simulink model "MatrixModel"  (R2018b)
settings: Solver=ode45  StartTime=0.0  StopTime=10.0  RelTol=1e-3  EnableMultiTasking=on
settings Model: Creator=sz609516  LastModifiedBy=fhu-eba
settings DataIOCC: LimitDataPoints=on  SaveFormat=Array
settings OptimizationCC: LifeSpan=inf
settings DebuggingCC: UnderspecifiedInitializationDetection=Classic  MergeDetectMultiDrivingBlocksExec=none  SolverPrmCheckMsg=warning  StateNameClashWarn=warning  SFUnexpectedBacktrackingDiag=warning  SFNoUnconditionalDefaultTransitionDiag=warning
settings HardwareCC: ProdBitPerPointer=32  ProdBitPerSizeT=32  ProdBitPerPtrDiffT=32  ProdLargestAtomicFloat=None  ProdIntDivRoundTo=Undefined  ProdEndianess=Unspecified  ProdWordSize=32  ProdHWDeviceType=32-bit Generic
settings ModelReferenceCC: PropagateSignalLabelsOutOfModel=off
settings SFSimCC: SimUseLocalCustomCode=off
settings RTWCC: RTWUseLocalCustomCode=off
settings CodeAppCC: StateflowObjectComments=on
settings GRTTargetCC: TargetLangStandard=C89/C90 (ANSI)  GeneratePreprocessorConditionals=Disable all
settings ConfigComp: CovMetricSettings=dw  CovHtmlReporting=on  CovSaveCumulativeToWorkspaceVar=on  CovSaveSingleToWorkspaceVar=on  CovExternalEMLEnable=off

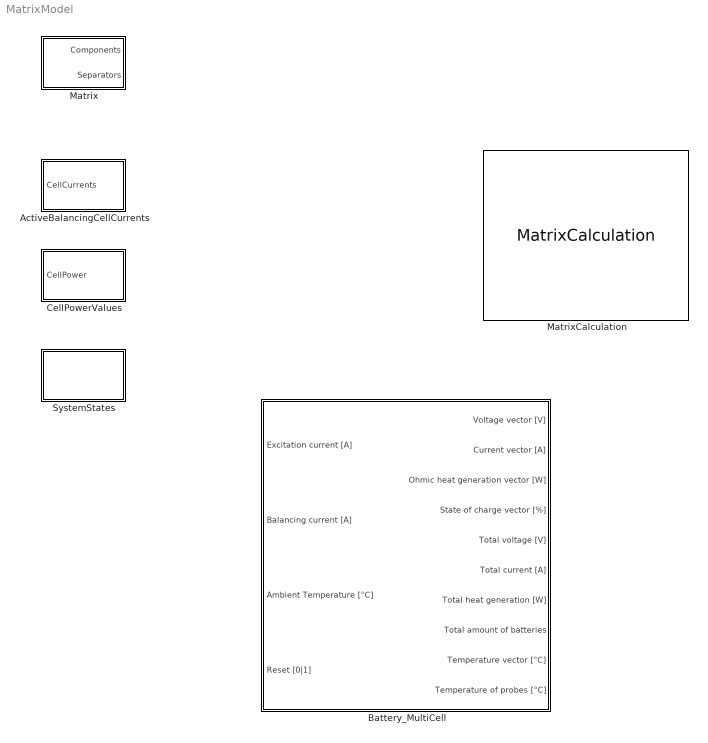
== system MatrixModel ==
  ActiveBalancingCellCurrents : Subsystem
  Battery_MultiCell : Subsystem
  CellPowerValues : Subsystem
  Matrix : Subsystem
  MatrixCalculation : S-Function  FunctionName=MatrixCalculation  SFunctionDeploymentMode=off  EnableBusSupport=off
  SystemStates : Subsystem

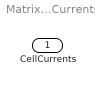
== system MatrixModel/ActiveBalancingCellCurrents ==
  CellCurrents : Inport

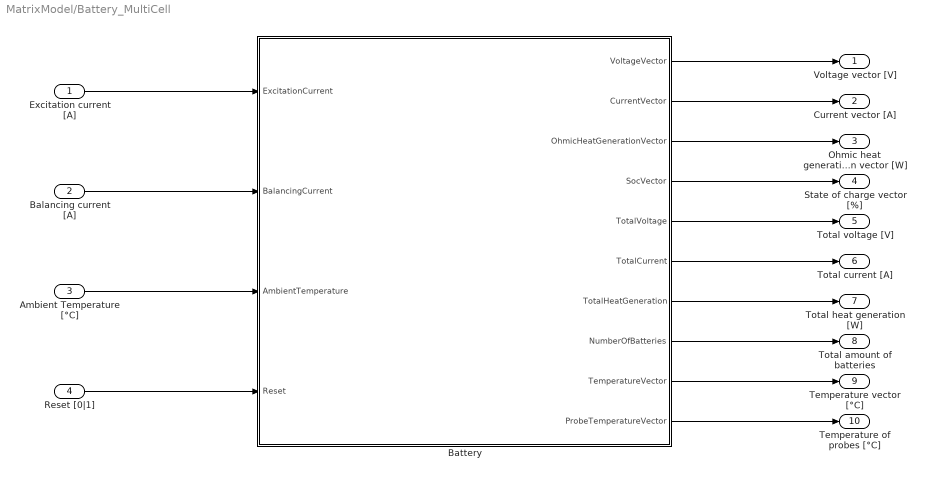
== system MatrixModel/Battery_MultiCell ==
  Excitation current [A] : Inport
  Balancing current [A] : Inport  Port=2
  Ambient Temperature [°C] : Inport  Port=3
  Reset [0|1] : Inport  Port=4
  Battery : Subsystem
  Voltage vector [V] : Outport
  Current vector [A] : Outport  Port=2
  Ohmic heat generation vector [W] : Outport  Port=3
  State of charge vector [%] : Outport  Port=4
  Total voltage [V] : Outport  Port=5
  Total current [A] : Outport  Port=6
  Total heat generation [W] : Outport  Port=7
  Total amount of batteries : Outport  Port=8
  Temperature vector [°C] : Outport  Port=9
  Temperature of probes [°C] : Outport  Port=10
  wires:
  Excitation current [A]/1 -> Battery/1(ExcitationCurrent)
  Balancing current [A]/1 -> Battery/2(BalancingCurrent)
  Ambient Temperature [°C]/1 -> Battery/3(AmbientTemperature)
  Reset [0|1]/1 -> Battery/4(Reset)
  Battery/1(VoltageVector) -> Voltage vector [V]/1
  Battery/2(CurrentVector) -> Current vector [A]/1
  Battery/3(OhmicHeatGenerationVector) -> Ohmic heat generation vector [W]/1
  Battery/4(SocVector) -> State of charge vector [%]/1
  Battery/5(TotalVoltage) -> Total voltage [V]/1
  Battery/6(TotalCurrent) -> Total current [A]/1
  Battery/7(TotalHeatGeneration) -> Total heat generation [W]/1
  Battery/8(NumberOfBatteries) -> Total amount of batteries/1
  Battery/9(TemperatureVector) -> Temperature vector [°C]/1
  Battery/10(ProbeTemperatureVector) -> Temperature of probes [°C]/1

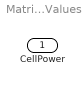
== system MatrixModel/CellPowerValues ==
  CellPower : Inport

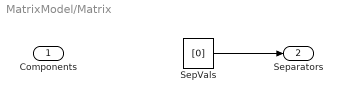
== system MatrixModel/Matrix ==
  SepVals : Constant  Value=[0]
  Components : Outport
  Separators : Outport  Port=2
  wires:
  SepVals/1 -> Separators/1

== system MatrixModel/SystemStates ==

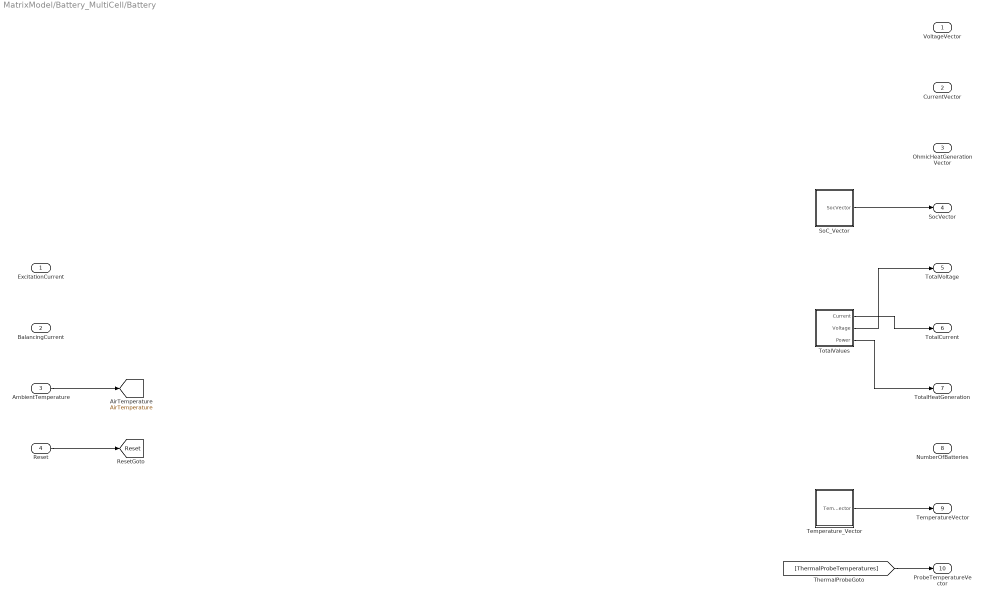
== system MatrixModel/Battery_MultiCell/Battery ==
  ExcitationCurrent : Inport
  BalancingCurrent : Inport  Port=2
  AmbientTemperature : Inport  Port=3
  Reset : Inport  Port=4
  SoC_Vector : Subsystem
  Temperature_Vector : Subsystem
  TotalValues : Subsystem
  VoltageVector : Outport
  CurrentVector : Outport  Port=2
  OhmicHeatGenerationVector : Outport  Port=3
  SocVector : Outport  Port=4
  TotalVoltage : Outport  Port=5
  TotalCurrent : Outport  Port=6
  TotalHeatGeneration : Outport  Port=7
  NumberOfBatteries : Outport  Port=8
  TemperatureVector : Outport  Port=9
  ProbeTemperatureVector : Outport  Port=10
  tag scope: AirTemperature=global, Reset=global
  wires:
  Temperature_Vector/1(TemperatureVector) -> TemperatureVector/1
  SoC_Vector/1(SocVector) -> SocVector/1
  TotalValues/1(Current) -> TotalCurrent/1
  TotalValues/3(Power) -> TotalHeatGeneration/1
  TotalValues/2(Voltage) -> TotalVoltage/1
  AmbientTemperature/1 -> [AirTemperature]
  Reset/1 -> [Reset]
  [ThermalProbeTemperatures] -> ProbeTemperatureVector/1

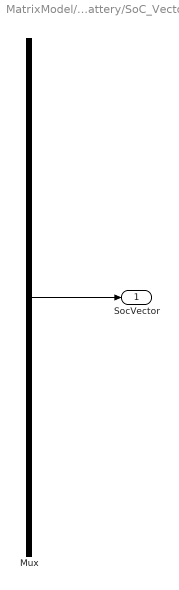
== system MatrixModel/Battery_MultiCell/Battery/SoC_Vector ==
  Mux : Mux  Inputs=3
  SocVector : Outport
  wires:
  Mux/1 -> SocVector/1

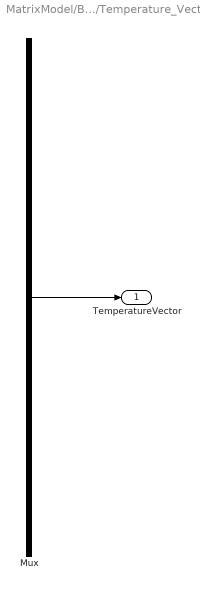
== system MatrixModel/Battery_MultiCell/Battery/Temperature_Vector ==
  Mux : Mux  Inputs=3
  TemperatureVector : Outport
  wires:
  Mux/1 -> TemperatureVector/1

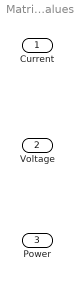
== system MatrixModel/Battery_MultiCell/Battery/TotalValues ==
  Current : Outport
  Voltage : Outport  Port=2
  Power : Outport  Port=3
